simulink model "insectDetectionSimulation"  (R2020b)
settings: Solver=FixedStepDiscrete  StartTime=0.0  StopTime=stopTime  RelTol=1e-3
PostLoadFcn:
  | loadDataSimulinkCallback
InitFcn:
  | initSimulinkModel
StopFcn:
  | verifySimulinkModel
values from neighbouring files (symbols this model uses):
  params = bestParams    [trainNet.m]
libraries: dspsrcs4 x1
settings Model: DataTypeOverride=Off  SimulationMode=rapid-accelerator  PauseTimes=1  Creator=trevor  LastModifiedBy=trevor
settings DataIOCC: SaveFormat=Array  SaveOutput=off  DSMLogging=off  SaveTime=off  ReturnWorkspaceOutputs=off
settings OptimizationCC: BlockReduction=off  ConditionallyExecuteInputs=off  DefaultParameterBehavior=Inlined
settings DebuggingCC: AlgebraicLoopMsg=error  SingleTaskRateTransMsg=error  SFMachineParentedDataDiag=error
settings HardwareCC: ProdBitPerPointer=32  ProdBitPerSizeT=32  ProdBitPerPtrDiffT=32  ProdLargestAtomicFloat=None  ProdIntDivRoundTo=Undefined  ProdEndianess=Unspecified  ProdWordSize=32  ProdHWDeviceType=ASIC/FPGA->ASIC/FPGA  TargetBitPerLong=64  TargetBitPerPointer=64  TargetBitPerSizeT=64  TargetBitPerPtrDiffT=64  TargetLongLongMode=on  TargetIntDivRoundTo=Zero  TargetEndianess=LittleEndian  TargetWordSize=64  TargetHWDeviceType=Custom Processor->MATLAB Host Computer  ProdEqTarget=off

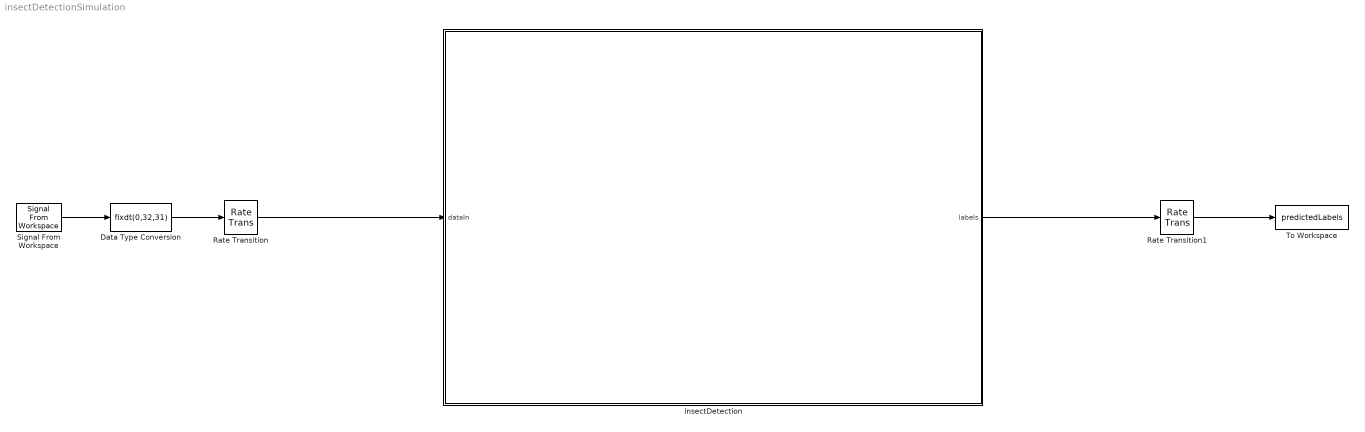
== system insectDetectionSimulation ==
  Data Type Conversion : DataTypeConversion  OutDataTypeStr=fixdt(0,32,31)
  Rate Transition : RateTransition  Deterministic=off  OutPortSampleTime=params.systemClockPeriod
  Rate Transition1 : RateTransition  Deterministic=off  OutPortSampleTime=params.samplingPeriod
  Signal From Workspace : dspsrcs4/Signal From Workspace  X=inputData  Ts=params.samplingPeriod  nsamps=1  OutputAfterFinalValue=Setting to zero  ignoreOrWarnInputAndFrameLengths=off  OutputFrames=off
  To Workspace : ToWorkspace  VariableName=predictedLabels  SampleTime=-1
      settings: Save2DSignal=2-D array (concatenate along first dimension)
  insectDetection : Subsystem
  wires:
  Signal From Workspace/1 -> Data Type Conversion/1
  Rate Transition1/1 -> To Workspace/1
  Rate Transition/1 -> insectDetection/1(dataIn)
  insectDetection/1(labels) -> Rate Transition1/1
  Data Type Conversion/1 -> Rate Transition/1

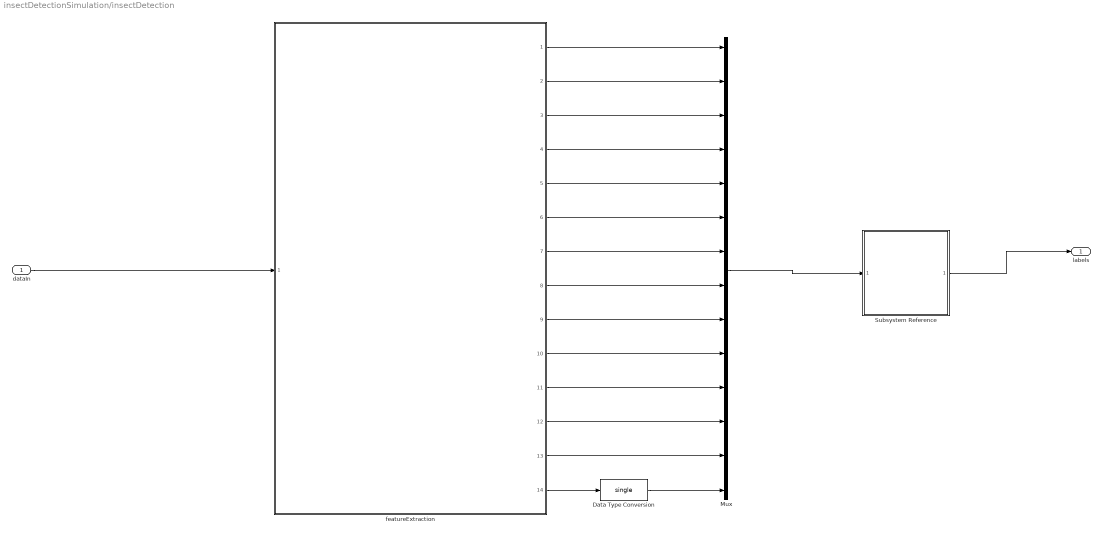
== system insectDetectionSimulation/insectDetection ==
  dataIn : Inport
  Data Type Conversion : DataTypeConversion  OutDataTypeStr=single  RndMeth=Nearest
  Mux : Mux  Inputs=14
  Subsystem Reference : Subsystem  ReferencedSubsystem=neuralNetInference
  featureExtraction : Subsystem  ReferencedSubsystem=featureExtraction
  labels : Outport
  wires:
  Subsystem Reference/1 -> labels/1
  Mux/1 -> Subsystem Reference/1
  dataIn/1 -> featureExtraction/1
  featureExtraction/1 -> Mux/1
  featureExtraction/2 -> Mux/2
  featureExtraction/3 -> Mux/3
  featureExtraction/4 -> Mux/4
  featureExtraction/5 -> Mux/5
  featureExtraction/6 -> Mux/6
  featureExtraction/7 -> Mux/7
  featureExtraction/8 -> Mux/8
  featureExtraction/9 -> Mux/9
  featureExtraction/10 -> Mux/10
  featureExtraction/11 -> Mux/11
  featureExtraction/12 -> Mux/12
  featureExtraction/13 -> Mux/13
  featureExtraction/14 -> Data Type Conversion/1
  Data Type Conversion/1 -> Mux/14
